simulink model "old_SMC"  (R2023a)
settings: Solver=FixedStepAuto  StartTime=0.0  StopTime=inf  RelTol=1e-3
undefined symbols (not defined in the file or in its folder): angular, linear
libraries: ros2lib x24
(part 1 of 2)

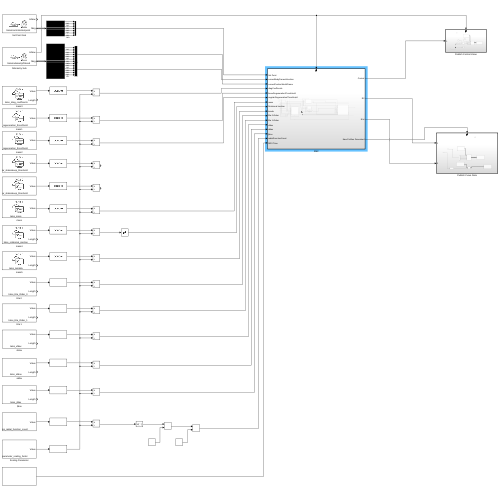
[thumbnail: Simulink's stored preview of the top-level diagram]
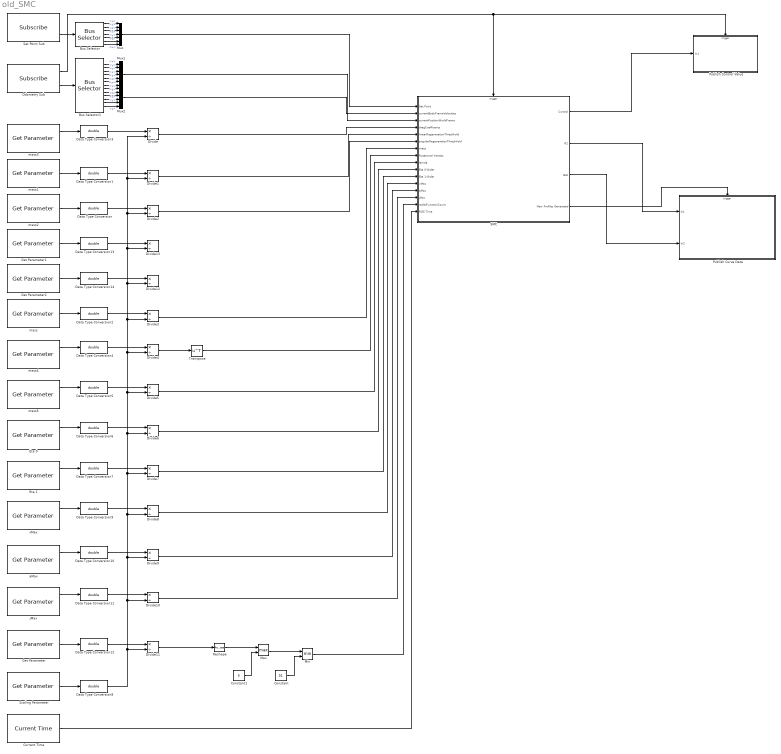
== system old_SMC ==
  Bus Selector : BusSelector  OutputSignals=position.x,position.y,position.z,orientation.x,orientation.y,orientation.z,orientation.w
  Bus Selector1 : BusSelector  OutputSignals=pose.pose.position.x,pose.pose.position.y,pose.pose.position.z,pose.pose.orientation.x,pose.pose.orientation.y,pose.pose.orientation.z,pose.pose.orientation.w,twist.twist.linear.x,twist.twist.linear.y,twist.twist.linear.z,twist.twist.angular.x,twist.twist.angular.y,twist.twist.angular.z
  Constant : Constant  Value=51
  Constant1 : Constant  Value=5
  Current Time : ros2lib/Current Time  OutputFormat=double  SampleTime=-1  ModelName=SMC
  Data Type Conversion{,1..14} (15 alike) : DataTypeConversion  OutDataTypeStr=double  SaturateOnIntegerOverflow=off  RndMeth=Floor
  Divide{,1..13} (14 alike) : Product  Inputs=*/
  Eta 0 : ros2lib/Get Parameter  ParameterName=talos_Eta_Order_0  ParameterType=int64[]  ParameterMaxArrayLength=6  ParameterInitialValue=0.0  SampleTime=-1  ModelName=SMC  BlockId=ParamGet_SMC_204
  Eta 1 : ros2lib/Get Parameter  ParameterName=talos_Eta_Order_1  ParameterType=int64[]  ParameterMaxArrayLength=6  ParameterInitialValue=0.0  SampleTime=-1  ModelName=SMC  BlockId=ParamGet_SMC_206
  Get Parameter : ros2lib/Get Parameter  ParameterName=talos_radial_function_count  ParameterType=int64  ParameterMaxArrayLength=16  ParameterInitialValue=0.0  SampleTime=-1  ModelName=SMC  BlockId=ParamGet_SMC_267
  Get Parameter1 : ros2lib/Get Parameter  ParameterName=talos_angular_stationkeep_threshold  ParameterType=int64  ParameterMaxArrayLength=16  ParameterInitialValue=0.0  SampleTime=-1  ModelName=SMC  BlockId=ParamGet_SMC_367
  Get Parameter2 : ros2lib/Get Parameter  ParameterName=talos_linear_stationkeep_threshold  ParameterType=int64  ParameterMaxArrayLength=16  ParameterInitialValue=0.0  SampleTime=-1  ModelName=SMC  BlockId=ParamGet_SMC_368
  Max : MinMax  Function=max  Inputs=2
  Min : MinMax  Inputs=2
  Mux : Mux  Inputs=7
  Mux1 : Mux  Inputs=7
  Mux2 : Mux  Inputs=6
  Odometry Sub : ros2lib/Subscribe  topicSource=Specify your own  topic=/talos/odometry/filtered  messageType=nav_msgs/Odometry  sampleTime=-1  QOSHistory=Keep last  QOSDepth=1  QOSReliability=Reliable  QOSDurability=Volatile
  Publish Control Value : Subsystem
  Publish Curve Data : Subsystem
  Reshape : Reshape  OutputDimensions=1
  SMC : Subsystem
  Scaling Parameter : ros2lib/Get Parameter  ParameterName=parameter_scaling_factor  ParameterType=int64  ParameterMaxArrayLength=16  ParameterInitialValue=1000000  SampleTime=-1  ModelName=SMC  BlockId=ParamGet_SMC_208
  Set Point Sub : ros2lib/Subscribe  topicSource=Specify your own  topic=/talos/controller/setpoint  messageType=geometry_msgs/Pose  sampleTime=-1  QOSHistory=Keep last  QOSDepth=1  QOSReliability=Reliable  QOSDurability=Volatile
  Transpose : Math  Operator=transpose
  aMax : ros2lib/Get Parameter  ParameterName=talos_aMax  ParameterType=int64[]  ParameterMaxArrayLength=6  ParameterInitialValue=0.0  SampleTime=-1  ModelName=SMC  BlockId=ParamGet_SMC_242
  jMax : ros2lib/Get Parameter  ParameterName=talos_jMax  ParameterType=int64[]  ParameterMaxArrayLength=6  ParameterInitialValue=0.0  SampleTime=-1  ModelName=SMC  BlockId=ParamGet_SMC_244
  mass : ros2lib/Get Parameter  ParameterName=talos_mass  ParameterType=int64  ParameterMaxArrayLength=16  ParameterInitialValue=0.0  SampleTime=-1  ModelName=SMC  BlockId=ParamGet_SMC_190
  mass1 : ros2lib/Get Parameter  ParameterName=talos_angular_regeneration_threshhold  ParameterType=int64  ParameterMaxArrayLength=16  ParameterInitialValue=0.0  SampleTime=-1  ModelName=SMC  BlockId=ParamGet_SMC_192
  mass2 : ros2lib/Get Parameter  ParameterName=talos_linear_regeneration_threshhold  ParameterType=int64  ParameterMaxArrayLength=16  ParameterInitialValue=0.0  SampleTime=-1  ModelName=SMC  BlockId=ParamGet_SMC_193
  mass3 : ros2lib/Get Parameter  ParameterName=talos_drag_coefficents  ParameterType=int64[]  ParameterMaxArrayLength=24  ParameterInitialValue=0.0  SampleTime=-1  ModelName=SMC  BlockId=ParamGet_SMC_197
  mass4 : ros2lib/Get Parameter  ParameterName=talos_rotational_inertias  ParameterType=int64[]  ParameterMaxArrayLength=3  ParameterInitialValue=0.0  SampleTime=-1  ModelName=SMC  BlockId=ParamGet_SMC_199
  mass5 : ros2lib/Get Parameter  ParameterName=talos_lambda  ParameterType=int64[]  ParameterMaxArrayLength=6  ParameterInitialValue=0.0  SampleTime=-1  ModelName=SMC  BlockId=ParamGet_SMC_202
  vMax : ros2lib/Get Parameter  ParameterName=talos_vMax  ParameterType=int64[]  ParameterMaxArrayLength=6  ParameterInitialValue=0.0  SampleTime=-1  ModelName=SMC  BlockId=ParamGet_SMC_240
  wires:
  Set Point Sub/2 -> Bus Selector/1
  Bus Selector/1 -> Mux/1  "<x>"
  Bus Selector/2 -> Mux/2  "<y>"
  Bus Selector/3 -> Mux/3  "<z>"
  Bus Selector/4 -> Mux/4  "<x>"
  Bus Selector/5 -> Mux/5  "<y>"
  Bus Selector/7 -> Mux/7  "<w>"
  Bus Selector/6 -> Mux/6  "<z>"
  Mux/1 -> SMC/1(Set Point)
  Odometry Sub/2 -> Bus Selector1/1
  Bus Selector1/1 -> Mux1/1  "<x>"
  Bus Selector1/2 -> Mux1/2  "<y>"
  Bus Selector1/3 -> Mux1/3  "<z>"
  Bus Selector1/4 -> Mux1/4  "<x>"
  Bus Selector1/5 -> Mux1/5  "<y>"
  Bus Selector1/6 -> Mux1/6  "<z>"
  Bus Selector1/7 -> Mux1/7  "<w>"
  Bus Selector1/8 -> Mux2/1  "<x>"
  Bus Selector1/9 -> Mux2/2  "<y>"
  Bus Selector1/10 -> Mux2/3  "<z>"
  Bus Selector1/11 -> Mux2/4  "<x>"
  Bus Selector1/12 -> Mux2/5  "<y>"
  Bus Selector1/13 -> Mux2/6  "<z>"
  Mux1/1 -> SMC/3(currentPositionWorldFrame)
  Mux2/1 -> SMC/2(currentBodyFrameVelocities)
  mass2/1 -> Data Type Conversion/1
  mass/1 -> Data Type Conversion2/1
  mass1/1 -> Data Type Conversion1/1
  mass3/1 -> Data Type Conversion3/1
  mass4/1 -> Data Type Conversion4/1
  mass5/1 -> Data Type Conversion5/1
  Eta 0/1 -> Data Type Conversion6/1
  Eta 1/1 -> Data Type Conversion7/1
  Scaling Parameter/1 -> Data Type Conversion8/1
  Data Type Conversion3/1 -> Divide/1
  Data Type Conversion1/1 -> Divide1/1
  Data Type Conversion/1 -> Divide2/1
  Data Type Conversion2/1 -> Divide3/1
  Data Type Conversion4/1 -> Divide4/1
  Data Type Conversion5/1 -> Divide5/1
  Data Type Conversion6/1 -> Divide6/1
  Data Type Conversion7/1 -> Divide7/1
  Data Type Conversion8/1 -> Divide11/2, Divide10/2, Divide9/2, Divide8/2, Divide7/2, Divide6/2, Divide5/2, Divide4/2, Divide3/2, Divide12/2, Divide13/2, Divide2/2, Divide1/2, Divide/2
  Divide/1 -> SMC/4(dragCoefficents)
  Divide1/1 -> SMC/5(linearRegenerationThreshhold)
  Divide2/1 -> SMC/6(angularRegenerationThreshhold)
  Divide3/1 -> SMC/7(mass)
  Divide4/1 -> Transpose/1
  Divide5/1 -> SMC/9(lamda)
  Divide6/1 -> SMC/10(Eta 0-Order)
  Divide7/1 -> SMC/11(Eta 1-Order)
  vMax/1 -> Data Type Conversion9/1
  aMax/1 -> Data Type Conversion10/1
  jMax/1 -> Data Type Conversion11/1
  Data Type Conversion9/1 -> Divide8/1
  Data Type Conversion10/1 -> Divide9/1
  Data Type Conversion11/1 -> Divide10/1
  Divide8/1 -> SMC/12(vMax)
  Divide9/1 -> SMC/13(aMax)
  Divide10/1 -> SMC/14(jMax)
  SMC/2(R2) -> Publish Curve Data/1(In1)
  SMC/3(tEst) -> Publish Curve Data/2(In2)
  SMC/4(New Profiles Generated) -> Publish Curve Data/Trigger
  Transpose/1 -> SMC/8(Rotational Inertias)
  Get Parameter/1 -> Data Type Conversion12/1
  Data Type Conversion12/1 -> Divide11/1
  Divide11/1 -> Reshape/1
  Constant/1 -> Min/2
  Min/1 -> SMC/15(radialFunctionCount)
  Current Time/1 -> SMC/16(ROS Time)
  Reshape/1 -> Max/1
  Max/1 -> Min/1
  Constant1/1 -> Max/2
  Get Parameter1/1 -> Data Type Conversion13/1
  Get Parameter2/1 -> Data Type Conversion14/1
  Data Type Conversion14/1 -> Divide12/1
  Data Type Conversion13/1 -> Divide13/1
  SMC/1(Control) -> Publish Control Value/1(In1)
  Odometry Sub/1 -> SMC/Trigger, Publish Control Value/Trigger

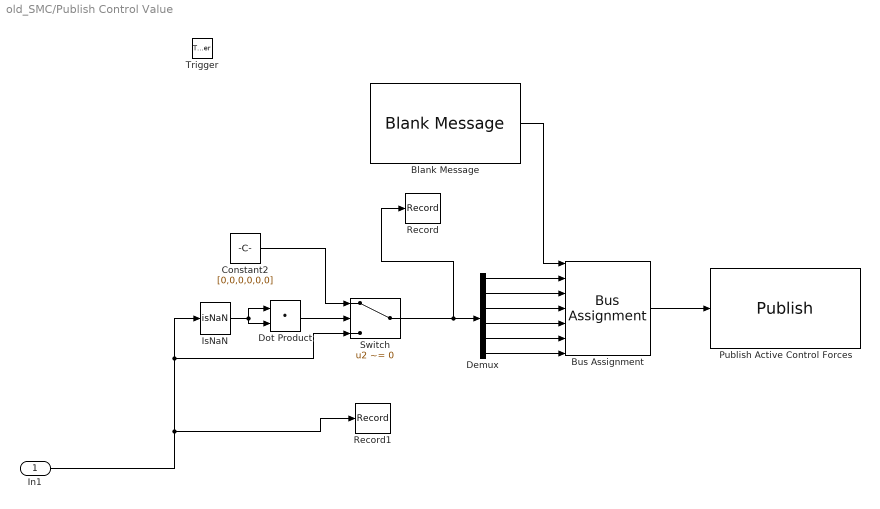
== system old_SMC/Publish Control Value ==
  In1 : Inport
  Trigger : TriggerPort  VariantControl=(inherit)  PortDimensions=1
  Blank Message : ros2lib/Blank Message  messageClass=Message  entityType=geometry_msgs/Twist  messageType=geometry_msgs/Twist  SampleTime=inf
  Bus Assignment : BusAssignment  AssignedSignals=linear.x,linear.y,linear.z,angular.x,angular.y,angular.z
  Constant2 : Constant  Value=[0,0,0,0,0,0]
  Demux : Demux  Outputs=6
  Dot Product : DotProduct  OutDataTypeStr=Inherit: Inherit via internal rule
  IsNaN : RelationalOperator  Operator=isNaN  OutDataTypeStr=boolean  RndMeth=Simplest  InputSameDT=off
  Publish Active Control Forces : ros2lib/Publish  topicSource=Specify your own  topic=/talos/controller/active_body_force  messageType=geometry_msgs/Twist  QOSHistory=Keep last  QOSDepth=1  QOSReliability=Reliable  QOSDurability=Volatile
  Record : Record  FileSettingsInternal="{\"entries\":[{\"content\":{\"excelSettings\":{\"content\":{},\"type\":\"Streamout.ExcelSettings\"}},\"type\":\"Streamout.FileSettingStorage\",\"uuid\":\"\"}],\"packageUris\":[\"http:\\/\\/schema.mathworks.com\\/mf0\\/streamout_blocks\\/R2020a\"],\"version\":\"1.0\"}"  Layout=[1 1]  SignalsInternal="{\"entries\":[{\"content\":{\"signals\":[{\"content\":{\"blockPath\":[],\"dimensions\":[6],\"domain\":\"\",\"hasChildren\":true,\"lineColor\":\"#d95319\",\"port\":1,\"sid\":[\"\"],\"signalID\":32364,\"signalName\":\"Switch\"},\"type\":\"RecordBlkView.Signal\",\"uuid\":\"\"},{\"content\":{\"blockPath\":[],\"channel\":[1],\"dimensions\":[6],\"domain\":\"\",\"lineColor\":\"#77ac30\",\"parentID\":32364,\"port\":1,\"sid\":[\"\"],\"signalID\":32365,\"signalName\":\"Switch\" ...(+1250 chars)"  VisualizationBindings="{\"sparklinesplugin\":{\"info\":[{\"bindingParametersList\":[],\"subplotID\":1}]}}"
  Record1 : Record  FileSettingsInternal="{\"entries\":[{\"content\":{\"excelSettings\":{\"content\":{},\"type\":\"Streamout.ExcelSettings\"}},\"type\":\"Streamout.FileSettingStorage\",\"uuid\":\"\"}],\"packageUris\":[\"http:\\/\\/schema.mathworks.com\\/mf0\\/streamout_blocks\\/R2020a\"],\"version\":\"1.0\"}"  Layout=[1 1]  SignalsInternal="{\"entries\":[{\"content\":{\"signals\":[{\"content\":{\"blockPath\":[],\"dimensions\":[6],\"domain\":\"\",\"hasChildren\":true,\"lineColor\":\"#7e2f8e\",\"port\":1,\"sid\":[\"\"],\"signalID\":32369,\"signalName\":\"In1\"},\"type\":\"RecordBlkView.Signal\",\"uuid\":\"\"},{\"content\":{\"blockPath\":[],\"channel\":[1],\"dimensions\":[6],\"domain\":\"\",\"lineColor\":\"#22b573\",\"parentID\":32369,\"plots\":[1],\"port\":1,\"sid\":[\"\"],\"signalID\":32370,\"signalName\" ...(+1289 chars)"  VisualizationBindings="{\"sparklinesplugin\":{\"info\":[{\"bindingParametersList\":[],\"subplotID\":1}]}}"
  Switch : Switch  Criteria=u2 ~= 0  SaturateOnIntegerOverflow=off  InputSameDT=off
  wires:
  Blank Message/1 -> Bus Assignment/1
  Switch/1 -> Record/1, Demux/1
  IsNaN/1 -> Dot Product/1, Dot Product/2
  Constant2/1 -> Switch/1
  Dot Product/1 -> Switch/2
  Demux/1 -> Bus Assignment/2
  Demux/2 -> Bus Assignment/3
  Demux/6 -> Bus Assignment/7
  Demux/3 -> Bus Assignment/4
  Demux/5 -> Bus Assignment/6
  In1/1 -> Record1/1, IsNaN/1, Switch/3
  Demux/4 -> Bus Assignment/5
  Bus Assignment/1 -> Publish Active Control Forces/1

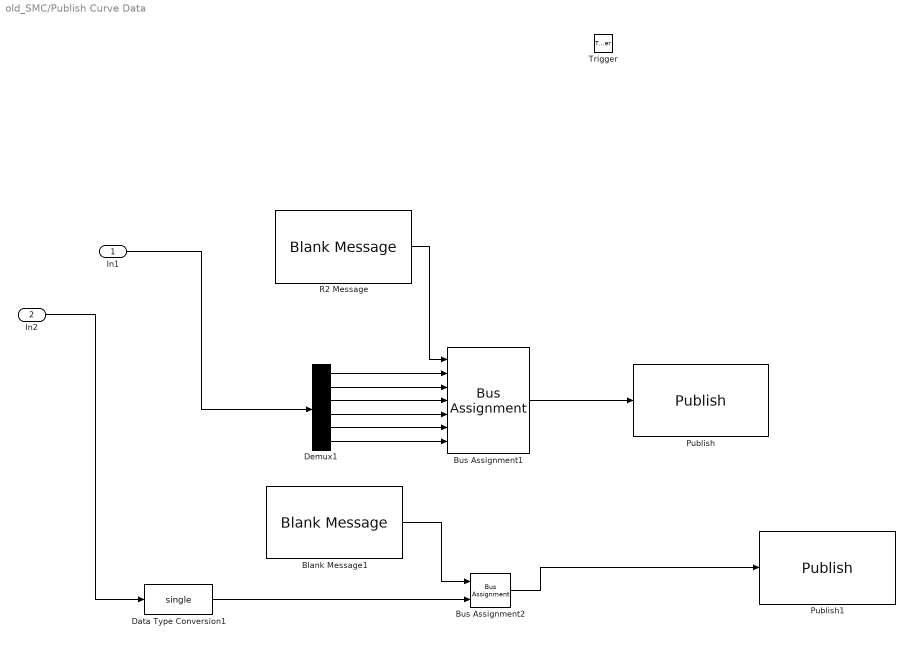
== system old_SMC/Publish Curve Data ==
  In1 : Inport
  In2 : Inport  Port=2
  Trigger : TriggerPort  VariantControl=(inherit)  PortDimensions=1
  Blank Message1 : ros2lib/Blank Message  messageClass=Message  entityType=std_msgs/Float32  messageType=std_msgs/Float32  SampleTime=inf
  Bus Assignment1 : BusAssignment  AssignedSignals=linear.x,angular.x,angular.y,angular.z,linear.y,linear.z
  Bus Assignment2 : BusAssignment  AssignedSignals=data
  Data Type Conversion1 : DataTypeConversion  OutDataTypeStr=single  SaturateOnIntegerOverflow=off  RndMeth=Floor
  Demux1 : Demux  Outputs=6
  Publish : ros2lib/Publish  topicSource=Specify your own  topic=/talos/controller/generatedR2  messageType=geometry_msgs/Twist  QOSHistory=Keep last  QOSDepth=1  QOSReliability=Reliable  QOSDurability=Volatile
  Publish1 : ros2lib/Publish  topicSource=Specify your own  topic=/talos/controller/curveTime  messageType=std_msgs/Float32  QOSHistory=Keep last  QOSDepth=1  QOSReliability=Reliable  QOSDurability=Volatile
  R2 Message : ros2lib/Blank Message  messageClass=Message  entityType=geometry_msgs/Twist  messageType=geometry_msgs/Twist  SampleTime=inf
  wires:
  Demux1/1 -> Bus Assignment1/2
  Demux1/6 -> Bus Assignment1/7
  Blank Message1/1 -> Bus Assignment2/1
  R2 Message/1 -> Bus Assignment1/1
  Demux1/5 -> Bus Assignment1/6
  Demux1/3 -> Bus Assignment1/4
  Demux1/4 -> Bus Assignment1/5
  Bus Assignment1/1 -> Publish/1
  In2/1 -> Data Type Conversion1/1
  Demux1/2 -> Bus Assignment1/3
  Bus Assignment2/1 -> Publish1/1
  In1/1 -> Demux1/1
  Data Type Conversion1/1 -> Bus Assignment2/2

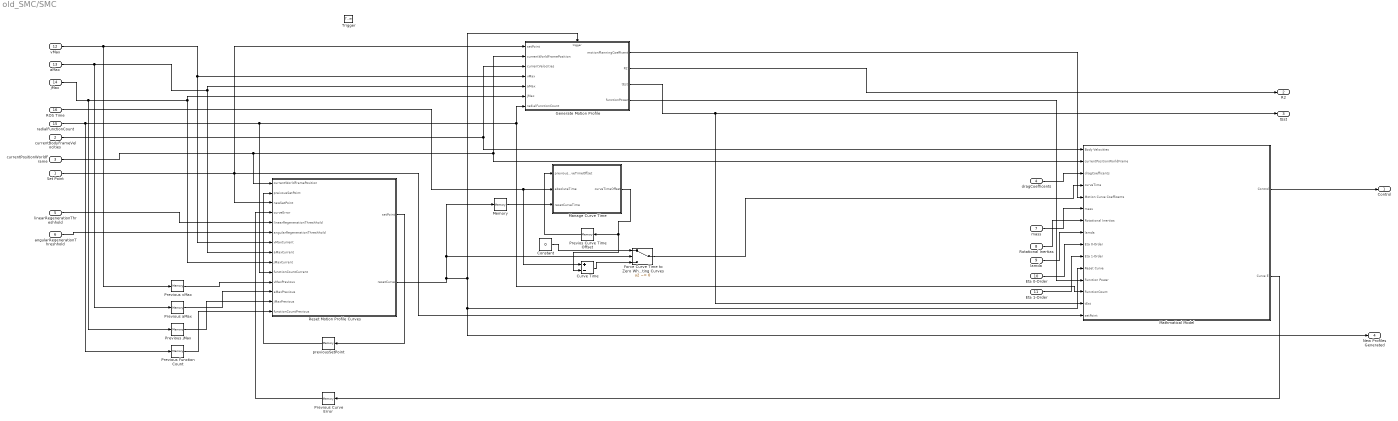
== system old_SMC/SMC ==
  Set Point : Inport
  currentBodyFrameVelocities : Inport  Port=2
  currentPositionWorldFrame : Inport  Port=3
  dragCoefficents : Inport  Port=4
  linearRegenerationThreshhold : Inport  Port=5
  angularRegenerationThreshhold : Inport  Port=6
  mass : Inport  Port=7
  Rotational Inertias : Inport  Port=8
  lamda : Inport  Port=9
  Eta 0-Order : Inport  Port=10
  Eta 1-Order : Inport  Port=11
  vMax : Inport  Port=12
  aMax : Inport  Port=13
  jMax : Inport  Port=14
  radialFunctionCount : Inport  Port=15
  ROS Time : Inport  Port=16
  Trigger : TriggerPort  VariantControl=(inherit)  PortDimensions=1
  Constant : Constant  Value=0
  Curve Time : Sum  Inputs=+-
  Force Curve Time to Zero When Reseting Curves : Switch  Criteria=u2 ~= 0  SaturateOnIntegerOverflow=off  InputSameDT=off
  Generate Motion Profile : Subsystem
  Manage Curve Time : MATLAB Function  TreatAsAtomicUnit=on
  Mathmatical Model : Subsystem
  Memory : Memory  InheritSampleTime=on
  Previos Curve Time Offset : Memory  InitialCondition=1700540270  InheritSampleTime=on
  Previous Curve Error : Memory  InheritSampleTime=on
  Previous Function Count : Memory  InheritSampleTime=on
  Previous aMax : Memory  InheritSampleTime=on
  Previous jMax : Memory  InheritSampleTime=on
  Previous vMax : Memory  InheritSampleTime=on
  Reset Motion Profile Curves : MATLAB Function  TreatAsAtomicUnit=on
  previousSetPoint : Memory  InheritSampleTime=on
  Control : Outport
  R2 : Outport  Port=2
  tEst : Outport  Port=3
  New Profiles Generated : Outport  Port=4
  wires:
  lamda/1 -> Mathmatical Model/8(lamda)
  currentPositionWorldFrame/1 -> Reset Motion Profile Curves/1(currentWorldFramePosition), Generate Motion Profile/2(currentWorldFramePosition), Mathmatical Model/2(currentPositionWorldFrame)
  mass/1 -> Mathmatical Model/6(mass)
  previousSetPoint/1 -> Reset Motion Profile Curves/2(preivousSetPoint)
  Mathmatical Model/2(Curve E) -> Previous Curve Error/1
  Rotational Inertias/1 -> Mathmatical Model/7(Rotational Inertias)
  currentBodyFrameVelocities/1 -> Generate Motion Profile/3(currentVelocities), Mathmatical Model/1(Body Velocities)
  Eta 0-Order/1 -> Mathmatical Model/9(Eta 0-Order)
  Eta 1-Order/1 -> Mathmatical Model/10(Eta 1-Order)
  dragCoefficents/1 -> Mathmatical Model/3(dragCoefficents)
  angularRegenerationThreshhold/1 -> Reset Motion Profile Curves/6(angularRegenerationThreshhold)
  linearRegenerationThreshhold/1 -> Reset Motion Profile Curves/5(linearRegenerationThreshhold)
  Previous Curve Error/1 -> Reset Motion Profile Curves/4(curveError)
  Reset Motion Profile Curves/1(setPoint) -> previousSetPoint/1
  Generate Motion Profile/1(motionPlanningCoefficents) -> Mathmatical Model/5(Motion Curve Coefficents)
  Generate Motion Profile/2(R2) -> R2/1
  Generate Motion Profile/3(tEst) -> Mathmatical Model/14(tEst), tEst/1
  vMax/1 -> Previous vMax/1, Reset Motion Profile Curves/7(vMaxCurrent), Generate Motion Profile/4(vMax)
  aMax/1 -> Previous aMax/1, Reset Motion Profile Curves/8(aMaxCurrent), Generate Motion Profile/5(aMax)
  jMax/1 -> Previous jMax/1, Reset Motion Profile Curves/9(jMaxCurrent), Generate Motion Profile/6(jMax)
  radialFunctionCount/1 -> Previous Function Count/1, Reset Motion Profile Curves/10(functionCountCurrent), Mathmatical Model/13(FunctionCount), Generate Motion Profile/7(radialFunctionCount)
  Generate Motion Profile/4(functionPower) -> Mathmatical Model/12(Function Power)
  Previous Function Count/1 -> Reset Motion Profile Curves/14(functionCountPrevious)
  Previous jMax/1 -> Reset Motion Profile Curves/13(jMaxPrevious)
  Previous aMax/1 -> Reset Motion Profile Curves/12(aMaxPrevious)
  Previous vMax/1 -> Reset Motion Profile Curves/11(vMaxPrevious)
  Reset Motion Profile Curves/2(resetCurve) -> Memory/1, Force Curve Time to Zero When Reseting Curves/2, New Profiles Generated/1, Mathmatical Model/11(Reset Curve), Generate Motion Profile/Trigger
  ROS Time/1 -> Curve Time/1, Manage Curve Time/2(absoluteTime)
  Manage Curve Time/1(curveTimeOffset) -> Curve Time/2, Previos Curve Time Offset/1
  Previos Curve Time Offset/1 -> Manage Curve Time/1(previousCurveTimeOffset)
  Memory/1 -> Manage Curve Time/3(resetCurveTime)
  Curve Time/1 -> Force Curve Time to Zero When Reseting Curves/3
  Force Curve Time to Zero When Reseting Curves/1 -> Mathmatical Model/4(curveTime)
  Constant/1 -> Force Curve Time to Zero When Reseting Curves/1
  Set Point/1 -> Mathmatical Model/15(setPoint), Reset Motion Profile Curves/3(newSetPoint), Generate Motion Profile/1(setPoint)
  Mathmatical Model/1(Control) -> Control/1

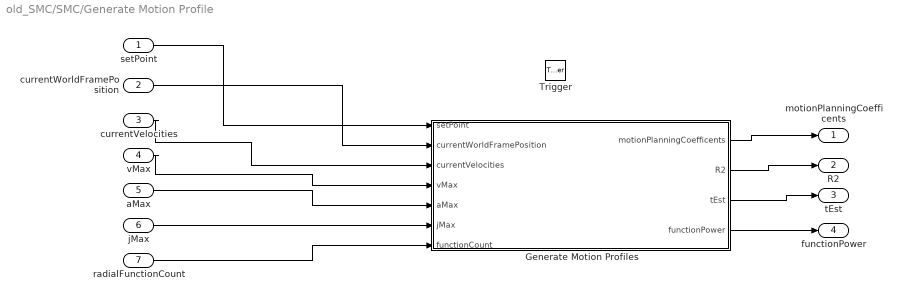
== system old_SMC/SMC/Generate Motion Profile ==
  setPoint : Inport
  currentWorldFramePosition : Inport  Port=2
  currentVelocities : Inport  Port=3
  vMax : Inport  Port=4
  aMax : Inport  Port=5
  jMax : Inport  Port=6
  radialFunctionCount : Inport  Port=7
  Trigger : TriggerPort  VariantControl=(inherit)  InitialTriggerSignalState=zero  PortDimensions=1
  Generate Motion Profiles : MATLAB Function  TreatAsAtomicUnit=on
  motionPlanningCoefficents : Outport
  R2 : Outport  Port=2
  tEst : Outport  Port=3
  functionPower : Outport  Port=4
  wires:
  Generate Motion Profiles/2(R2) -> R2/1
  currentVelocities/1 -> Generate Motion Profiles/3(currentVelocities)
  Generate Motion Profiles/1(motionPlanningCoefficents) -> motionPlanningCoefficents/1
  Generate Motion Profiles/3(tEst) -> tEst/1
  setPoint/1 -> Generate Motion Profiles/1(setPoint)
  aMax/1 -> Generate Motion Profiles/5(aMax)
  vMax/1 -> Generate Motion Profiles/4(vMax)
  currentWorldFramePosition/1 -> Generate Motion Profiles/2(currentWorldFramePosition)
  jMax/1 -> Generate Motion Profiles/6(jMax)
  radialFunctionCount/1 -> Generate Motion Profiles/7(functionCount)
  Generate Motion Profiles/4(functionPower) -> functionPower/1

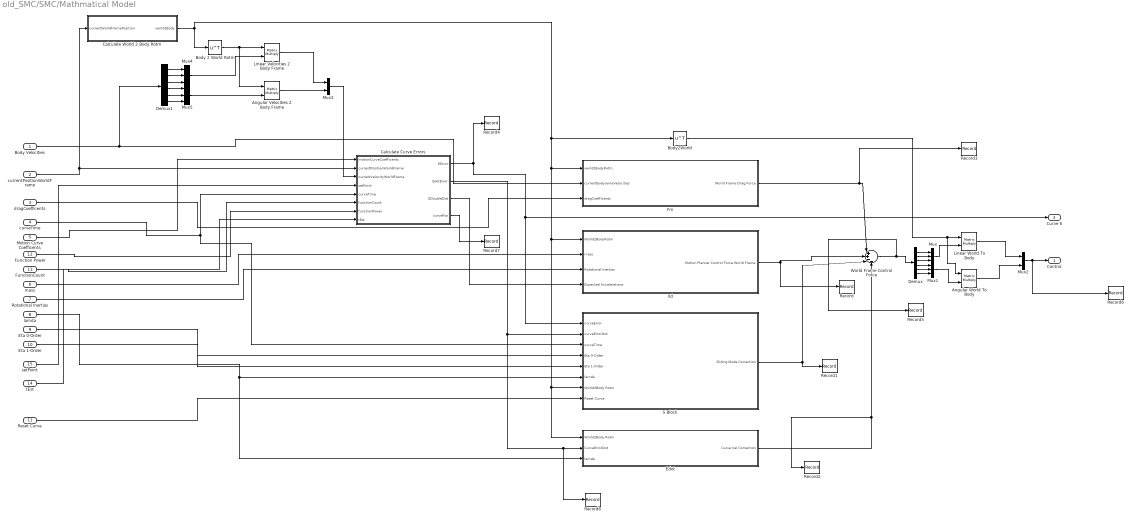
== system old_SMC/SMC/Mathmatical Model ==
  Body Velocities : Inport
  currentPositionWorldFrame : Inport  Port=2
  dragCoefficents : Inport  Port=3
  curveTime : Inport  Port=4
  Motion Curve Coefficents : Inport  Port=5
  mass : Inport  Port=6
  Rotational Inertias : Inport  Port=7
  lamda : Inport  Port=8
  Eta 0-Order : Inport  Port=9
  Eta 1-Order : Inport  Port=10
  Reset Curve : Inport  Port=11
  Function Power : Inport  Port=12
  FunctionCount : Inport  Port=13
  tEst : Inport  Port=14
  setPoint : Inport  Port=15
  Angular Velocities 2 Body Frame : Product  Multiplication=Matrix(*)
  Angular World To Body : Product  Multiplication=Matrix(*)
  Body 2 World Rotm : Math  Operator=transpose
  Body2World : Math  Operator=transpose
  Calculate Curve Errors : MATLAB Function  TreatAsAtomicUnit=on
  Calculate World 2 Body Rotm : MATLAB Function  TreatAsAtomicUnit=on
  Demux : Demux  Outputs=6
  Demux1 : Demux  Outputs=6
  Edot : Subsystem
  Fm : Subsystem
  Linear Velocities 2 Body Frame : Product  Multiplication=Matrix(*)
  Linear World To Body : Product  Multiplication=Matrix(*)
  Mux{,1,4..5} (4 alike) : Mux  Inputs=3
  Mux2 : Mux  Inputs=2
  Mux3 : Mux  Inputs=2
  Record : Record  FileSettingsInternal="{\"entries\":[{\"content\":{\"excelSettings\":{\"content\":{},\"type\":\"Streamout.ExcelSettings\"}},\"type\":\"Streamout.FileSettingStorage\",\"uuid\":\"\"}],\"packageUris\":[\"http:\\/\\/schema.mathworks.com\\/mf0\\/streamout_blocks\\/R2020a\"],\"version\":\"1.0\"}"  Layout=[1 1]  SignalsInternal="{\"entries\":[{\"content\":{\"signals\":[{\"content\":{\"blockPath\":[],\"dimensions\":[6,1],\"domain\":\"\",\"hasChildren\":true,\"lineColor\":\"#139fff\",\"port\":1,\"sid\":[\"\"],\"signalID\":32309,\"signalName\":\"Xd\"},\"type\":\"RecordBlkView.Signal\",\"uuid\":\"\"},{\"content\":{\"blockPath\":[],\"channel\":[1,1],\"dimensions\":[6,1],\"domain\":\"\",\"lineColor\":\"#fe330a\",\"parentID\":32309,\"plots\":[1],\"port\":1,\"sid\":[\"\"],\"signalID\":32310,\"signal ...(+1308 chars)"  VisualizationBindings="{\"sparklinesplugin\":{\"info\":[{\"bindingParametersList\":[],\"subplotID\":1}]}}"
  Record1 : Record  FileSettingsInternal="{\"entries\":[{\"content\":{\"excelSettings\":{\"content\":{},\"type\":\"Streamout.ExcelSettings\"}},\"type\":\"Streamout.FileSettingStorage\",\"uuid\":\"\"}],\"packageUris\":[\"http:\\/\\/schema.mathworks.com\\/mf0\\/streamout_blocks\\/R2020a\"],\"version\":\"1.0\"}"  Layout=[1 1]  SignalsInternal="{\"entries\":[{\"content\":{\"signals\":[{\"content\":{\"blockPath\":[],\"dimensions\":[6,1],\"domain\":\"\",\"hasChildren\":true,\"lineColor\":\"#b746ff\",\"port\":1,\"sid\":[\"\"],\"signalID\":32314,\"signalName\":\"S Block\"},\"type\":\"RecordBlkView.Signal\",\"uuid\":\"\"},{\"content\":{\"blockPath\":[],\"channel\":[1,1],\"dimensions\":[6,1],\"domain\":\"\",\"lineColor\":\"#0072bd\",\"parentID\":32314,\"plots\":[1],\"port\":1,\"sid\":[\"\"],\"signalID\":32315,\"s ...(+1343 chars)"  VisualizationBindings="{\"sparklinesplugin\":{\"info\":[{\"bindingParametersList\":[],\"subplotID\":1}]}}"
  Record2 : Record  FileSettingsInternal="{\"entries\":[{\"content\":{\"excelSettings\":{\"content\":{},\"type\":\"Streamout.ExcelSettings\"}},\"type\":\"Streamout.FileSettingStorage\",\"uuid\":\"\"}],\"packageUris\":[\"http:\\/\\/schema.mathworks.com\\/mf0\\/streamout_blocks\\/R2020a\"],\"version\":\"1.0\"}"  Layout=[1 1]  SignalsInternal="{\"entries\":[{\"content\":{\"signals\":[{\"content\":{\"blockPath\":[],\"dimensions\":[6,1],\"domain\":\"\",\"hasChildren\":true,\"lineColor\":\"#ff13a6\",\"port\":1,\"sid\":[\"\"],\"signalID\":32319,\"signalName\":\"Edot\"},\"type\":\"RecordBlkView.Signal\",\"uuid\":\"\"},{\"content\":{\"blockPath\":[],\"channel\":[1,1],\"dimensions\":[6,1],\"domain\":\"\",\"lineColor\":\"#edb120\",\"parentID\":32319,\"port\":1,\"sid\":[\"\"],\"signalID\":32320,\"signalName\":\"Edo ...(+1298 chars)"  VisualizationBindings="{\"sparklinesplugin\":{\"info\":[{\"bindingParametersList\":[],\"subplotID\":1}]}}"
  Record3 : Record  FileSettingsInternal="{\"entries\":[{\"content\":{\"excelSettings\":{\"content\":{},\"type\":\"Streamout.ExcelSettings\"}},\"type\":\"Streamout.FileSettingStorage\",\"uuid\":\"\"}],\"packageUris\":[\"http:\\/\\/schema.mathworks.com\\/mf0\\/streamout_blocks\\/R2020a\"],\"version\":\"1.0\"}"  Layout=[1 1]  SignalsInternal="{\"entries\":[{\"content\":{\"signals\":[{\"content\":{\"blockPath\":[],\"dimensions\":[6],\"domain\":\"\",\"hasChildren\":true,\"lineColor\":\"#22b573\",\"port\":1,\"sid\":[\"\"],\"signalID\":32324,\"signalName\":\"Fm\"},\"type\":\"RecordBlkView.Signal\",\"uuid\":\"\"},{\"content\":{\"blockPath\":[],\"channel\":[1],\"dimensions\":[6],\"domain\":\"\",\"lineColor\":\"#77ac30\",\"parentID\":32324,\"plots\":[1],\"port\":1,\"sid\":[\"\"],\"signalID\":32325,\"signalName\": ...(+1246 chars)"  VisualizationBindings="{\"sparklinesplugin\":{\"info\":[{\"bindingParametersList\":[],\"subplotID\":1}]}}"
  Record4 : Record  FileSettingsInternal="{\"entries\":[{\"content\":{\"excelSettings\":{\"content\":{},\"type\":\"Streamout.ExcelSettings\"}},\"type\":\"Streamout.FileSettingStorage\",\"uuid\":\"\"}],\"packageUris\":[\"http:\\/\\/schema.mathworks.com\\/mf0\\/streamout_blocks\\/R2020a\"],\"version\":\"1.0\"}"  Layout=[1 1]  SignalsInternal="{\"entries\":[{\"content\":{\"signals\":[{\"content\":{\"blockPath\":[],\"dimensions\":[6,1],\"domain\":\"\",\"hasChildren\":true,\"lineColor\":\"#d95319\",\"port\":1,\"sid\":[\"\"],\"signalID\":32329,\"signalName\":\"Calculate Curve Errors:1\"},\"type\":\"RecordBlkView.Signal\",\"uuid\":\"\"},{\"content\":{\"blockPath\":[],\"channel\":[1,1],\"dimensions\":[6,1],\"domain\":\"\",\"lineColor\":\"#a2142f\",\"parentID\":32329,\"plots\":[1],\"port\":1,\"sid\":[\"\"],\"s ...(+1462 chars)"  VisualizationBindings="{\"sparklinesplugin\":{\"info\":[{\"bindingParametersList\":[],\"subplotID\":1}]}}"
  Record5 : Record  FileSettingsInternal="{\"entries\":[{\"content\":{\"excelSettings\":{\"content\":{},\"type\":\"Streamout.ExcelSettings\"}},\"type\":\"Streamout.FileSettingStorage\",\"uuid\":\"\"}],\"packageUris\":[\"http:\\/\\/schema.mathworks.com\\/mf0\\/streamout_blocks\\/R2020a\"],\"version\":\"1.0\"}"  Layout=[1 1]  SignalsInternal="{\"entries\":[{\"content\":{\"signals\":[{\"content\":{\"blockPath\":[],\"dimensions\":[6,1],\"domain\":\"\",\"hasChildren\":true,\"lineColor\":\"#7e2f8e\",\"port\":1,\"sid\":[\"\"],\"signalID\":32334,\"signalName\":\"World Frame Control Force\"},\"type\":\"RecordBlkView.Signal\",\"uuid\":\"\"},{\"content\":{\"blockPath\":[],\"channel\":[1,1],\"dimensions\":[6,1],\"domain\":\"\",\"lineColor\":\"#4dbeee\",\"parentID\":32334,\"port\":1,\"sid\":[\"\"],\"signalID\":32 ...(+1409 chars)"  VisualizationBindings="{\"sparklinesplugin\":{\"info\":[{\"bindingParametersList\":[],\"subplotID\":1}]}}"
  Record6 : Record  FileSettingsInternal="{\"entries\":[{\"content\":{\"excelSettings\":{\"content\":{},\"type\":\"Streamout.ExcelSettings\"}},\"type\":\"Streamout.FileSettingStorage\",\"uuid\":\"\"}],\"packageUris\":[\"http:\\/\\/schema.mathworks.com\\/mf0\\/streamout_blocks\\/R2020a\"],\"version\":\"1.0\"}"  Layout=[1 1]  SignalsInternal="{\"entries\":[{\"content\":{\"signals\":[{\"content\":{\"blockPath\":[],\"dimensions\":[6],\"domain\":\"\",\"hasChildren\":true,\"lineColor\":\"#4dbeee\",\"port\":1,\"sid\":[\"\"],\"signalID\":32339,\"signalName\":\"Mux2\"},\"type\":\"RecordBlkView.Signal\",\"uuid\":\"\"},{\"content\":{\"blockPath\":[],\"channel\":[1],\"dimensions\":[6],\"domain\":\"\",\"lineColor\":\"#0072bd\",\"parentID\":32339,\"port\":1,\"sid\":[\"\"],\"signalID\":32340,\"signalName\":\"Mux2\"},\"t ...(+1236 chars)"  VisualizationBindings="{\"sparklinesplugin\":{\"info\":[{\"bindingParametersList\":[],\"subplotID\":1}]}}"
  Record7 : Record  FileSettingsInternal="{\"entries\":[{\"content\":{\"excelSettings\":{\"content\":{},\"type\":\"Streamout.ExcelSettings\"}},\"type\":\"Streamout.FileSettingStorage\",\"uuid\":\"\"}],\"packageUris\":[\"http:\\/\\/schema.mathworks.com\\/mf0\\/streamout_blocks\\/R2020a\"],\"version\":\"1.0\"}"  Layout=[1 1]  SignalsInternal="{\"entries\":[{\"content\":{\"signals\":[{\"content\":{\"blockPath\":[],\"dimensions\":[6,1],\"domain\":\"\",\"hasChildren\":true,\"lineColor\":\"#139fff\",\"port\":1,\"sid\":[\"\"],\"signalID\":32344,\"signalName\":\"Calculate Curve Errors:4\"},\"type\":\"RecordBlkView.Signal\",\"uuid\":\"\"},{\"content\":{\"blockPath\":[],\"channel\":[1,1],\"dimensions\":[6,1],\"domain\":\"\",\"lineColor\":\"#d95319\",\"parentID\":32344,\"port\":1,\"sid\":[\"\"],\"signalID\":323 ...(+1402 chars)"  VisualizationBindings="{\"sparklinesplugin\":{\"info\":[{\"bindingParametersList\":[],\"subplotID\":1}]}}"
  Record8 : Record  FileSettingsInternal="{\"entries\":[{\"content\":{\"excelSettings\":{\"content\":{},\"type\":\"Streamout.ExcelSettings\"}},\"type\":\"Streamout.FileSettingStorage\",\"uuid\":\"\"}],\"packageUris\":[\"http:\\/\\/schema.mathworks.com\\/mf0\\/streamout_blocks\\/R2020a\"],\"version\":\"1.0\"}"  Layout=[1 1]  SignalsInternal="{\"entries\":[{\"content\":{\"signals\":[{\"content\":{\"blockPath\":[],\"dimensions\":[6,1],\"domain\":\"\",\"hasChildren\":true,\"lineColor\":\"#b746ff\",\"port\":1,\"sid\":[\"\"],\"signalID\":32349,\"signalName\":\"Calculate Curve Errors:2\"},\"type\":\"RecordBlkView.Signal\",\"uuid\":\"\"},{\"content\":{\"blockPath\":[],\"channel\":[1,1],\"dimensions\":[6,1],\"domain\":\"\",\"lineColor\":\"#7e2f8e\",\"parentID\":32349,\"port\":1,\"sid\":[\"\"],\"signalID\":323 ...(+1402 chars)"  VisualizationBindings="{\"sparklinesplugin\":{\"info\":[{\"bindingParametersList\":[],\"subplotID\":1}]}}"
  S Block : Subsystem
  World Frame Control Force : Sum  Inputs=|++--
  Xd : Subsystem
  Control : Outport
  Curve E : Outport  Port=2
  wires:
  Reset Curve/1 -> S Block/8(Reset Curve)
  Eta 0-Order/1 -> S Block/4(Eta 0-Order)
  Eta 1-Order/1 -> S Block/5(Eta 1-Order)
  Body Velocities/1 -> Demux1/1, Fm/2(currentBodyrameVelocities)
  Calculate Curve Errors/2(EdotError) -> Record8/1, Edot/2(CurveErrorDot), S Block/2(curveErrorDot)
  mass/1 -> Xd/2(mass)
  Motion Curve Coefficents/1 -> Calculate Curve Errors/1(motionCurveCoefficents)
  currentPositionWorldFrame/1 -> Calculate World 2 Body Rotm/1(currentWorldFramePosition), Calculate Curve Errors/2(currentPositionWorldFrame)
  curveTime/1 -> Calculate Curve Errors/5(curveTime), S Block/3(curveTime)
  Xd/1(Motion Planner Control Force World Frame) -> World Frame Control Force/2, Record/1
  Calculate Curve Errors/1(EError) -> Curve E/1, S Block/1(curveError), Record4/1
  S Block/1("Sliding Mode Correction ") -> World Frame Control Force/3, Record1/1
  lamda/1 -> Edot/3(lamda), S Block/6(lamda)
  Rotational Inertias/1 -> Xd/3(Rotational Inertias)
  Calculate World 2 Body Rotm/1(world2Body) -> Body 2 World Rotm/1, Body2World/1, Edot/1(World2Body Rotm), S Block/7(World2Body Rotm), Xd/1(World2BodyRotm), Fm/1(world2BodyRotm)
  Edot/1(Curve Vel Correction) -> World Frame Control Force/4, Record2/1
  World Frame Control Force/1 -> Record5/1, Demux/1
  Demux/1 -> Mux/1
  Demux/2 -> Mux/2
  Demux/3 -> Mux/3
  Demux/6 -> Mux1/3
  Demux/5 -> Mux1/2
  Demux/4 -> Mux1/1
  Mux/1 -> Linear World To Body/2
  Mux1/1 -> Angular World To Body/2
  Linear World To Body/1 -> Mux2/1
  Angular World To Body/1 -> Mux2/2
  Mux2/1 -> Record6/1, Control/1
  Body2World/1 -> Angular World To Body/1, Linear World To Body/1
  Function Power/1 -> Calculate Curve Errors/7(functionPower)
  FunctionCount/1 -> Calculate Curve Errors/6(functionCount)
  tEst/1 -> Calculate Curve Errors/8(tEst)
  dragCoefficents/1 -> Fm/3(dragCoefficents)
  Body 2 World Rotm/1 -> Angular Velocities 2 Body Frame/1, Linear Velocities 2 Body Frame/1
  Linear Velocities 2 Body Frame/1 -> Mux3/1
  Angular Velocities 2 Body Frame/1 -> Mux3/2
  Mux3/1 -> Calculate Curve Errors/3(currentVelocityWorldFrame)
  Mux4/1 -> Linear Velocities 2 Body Frame/2
  Demux1/2 -> Mux4/2
  Demux1/1 -> Mux4/1
  Demux1/3 -> Mux4/3
  Demux1/5 -> Mux5/2
  Demux1/4 -> Mux5/1
  Demux1/6 -> Mux5/3
  Mux5/1 -> Angular Velocities 2 Body Frame/2
  setPoint/1 -> Calculate Curve Errors/4(setPoint)
  Fm/1(World Frame Drag Force) -> Record3/1, World Frame Control Force/1
  Calculate Curve Errors/3(EDoubleDot) -> Xd/4(Expected Accelerations)
  Calculate Curve Errors/4(curvePos) -> Record7/1

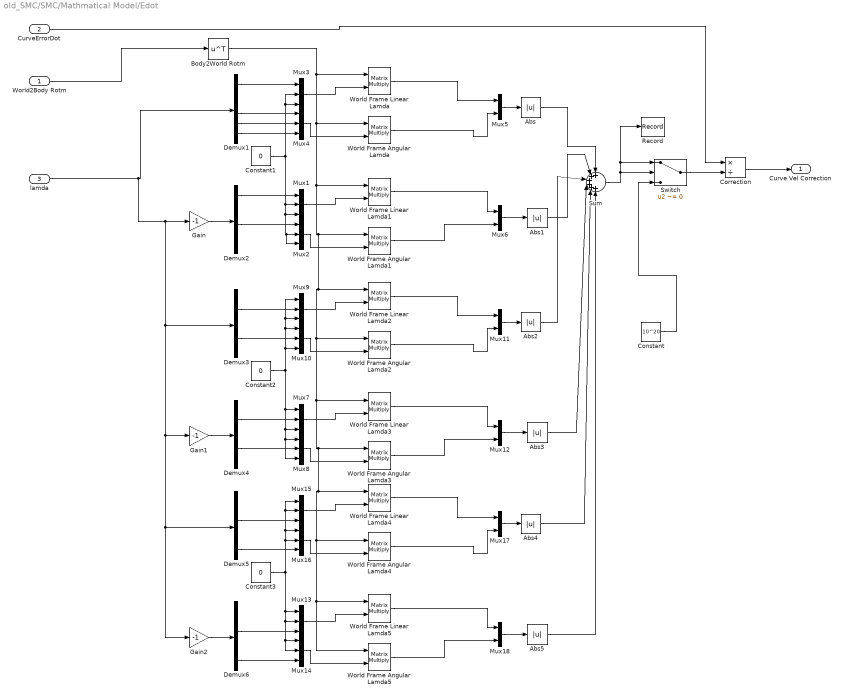
== system old_SMC/SMC/Mathmatical Model/Edot ==
  World2Body Rotm : Inport
  CurveErrorDot : Inport  Port=2
  lamda : Inport  Port=3
  Abs{,1..5} (6 alike) : Abs  SaturateOnIntegerOverflow=off
  Body2World Rotm : Math  Operator=transpose
  Constant : Constant  Value=10^20
  Constant1 : Constant  Value=0
  Constant2 : Constant  Value=0
  Constant3 : Constant  Value=0
  Correction : Product  Inputs=*/
  Demux{1..6} (6 alike) : Demux  Outputs=6
  Gain : Gain  Gain=-1
  Gain1 : Gain  Gain=-1
  Gain2 : Gain  Gain=-1
  Mux{1..4,7..10,13..16} (12 alike) : Mux  Inputs=3
  Mux{5..6,11..12,17..18} (6 alike) : Mux  Inputs=2
  Record : Record  FileSettingsInternal="{\"entries\":[{\"content\":{\"excelSettings\":{\"content\":{},\"type\":\"Streamout.ExcelSettings\"}},\"type\":\"Streamout.FileSettingStorage\",\"uuid\":\"\"}],\"packageUris\":[\"http:\\/\\/schema.mathworks.com\\/mf0\\/streamout_blocks\\/R2020a\"],\"version\":\"1.0\"}"  Layout=[1 1]  SignalsInternal="{\"entries\":[{\"content\":{\"signals\":[{\"content\":{\"blockPath\":[],\"dimensions\":[6],\"domain\":\"\",\"hasChildren\":true,\"lineColor\":\"#ff13a6\",\"port\":1,\"sid\":[\"\"],\"signalID\":32354,\"signalName\":\"Sum\"},\"type\":\"RecordBlkView.Signal\",\"uuid\":\"\"},{\"content\":{\"blockPath\":[],\"channel\":[1],\"dimensions\":[6],\"domain\":\"\",\"lineColor\":\"#4dbeee\",\"parentID\":32354,\"plots\":[1],\"port\":1,\"sid\":[\"\"],\"signalID\":32355,\"signalName\" ...(+1253 chars)"  VisualizationBindings="{\"sparklinesplugin\":{\"info\":[{\"bindingParametersList\":[],\"subplotID\":1}]}}"
  Sum : Sum  Inputs=++++++
  Switch : Switch  Criteria=u2 ~= 0  SaturateOnIntegerOverflow=off  InputSameDT=off
  World Frame Angular Lamda{,1..5} (6 alike) : Product  Multiplication=Matrix(*)
  World Frame Linear Lamda{,1..5} (6 alike) : Product  Multiplication=Matrix(*)
  Curve Vel Correction : Outport
  wires:
  Mux3/1 -> World Frame Linear Lamda/2
  CurveErrorDot/1 -> Correction/1
  World2Body Rotm/1 -> Body2World Rotm/1
  Mux4/1 -> World Frame Angular Lamda/2
  Demux1/4 -> Mux4/1
  Correction/1 -> Curve Vel Correction/1
  Demux1/1 -> Mux3/1
  Switch/1 -> Correction/2
  Constant/1 -> Switch/3
  Mux6/1 -> Abs1/1
  Sum/1 -> Record/1, Switch/1, Switch/2
  Mux5/1 -> Abs/1
  World Frame Linear Lamda/1 -> Mux5/1
  World Frame Angular Lamda/1 -> Mux5/2
  Demux2/1 -> Mux1/1
  Mux2/1 -> World Frame Angular Lamda1/2
  Mux1/1 -> World Frame Linear Lamda1/2
  World Frame Angular Lamda1/1 -> Mux6/2
  World Frame Linear Lamda1/1 -> Mux6/1
  Demux2/4 -> Mux2/1
  Demux1/5 -> Mux4/2
  Demux1/6 -> Mux4/3
  Gain/1 -> Demux2/1
  Constant1/1 -> Mux3/3, Mux3/2, Mux2/3, Mux2/2, Mux1/3, Mux1/2
  Abs/1 -> Sum/1
  Abs1/1 -> Sum/2
  Mux10/1 -> World Frame Angular Lamda2/2
  Mux8/1 -> World Frame Angular Lamda3/2
  World Frame Angular Lamda2/1 -> Mux11/2
  World Frame Angular Lamda3/1 -> Mux12/2
  Mux11/1 -> Abs2/1
  Constant2/1 -> Mux10/3, Mux10/1, Mux9/1, Mux9/3, Mux7/1, Mux8/3, Mux8/1, Mux7/3
  World Frame Linear Lamda3/1 -> Mux12/1
  Mux7/1 -> World Frame Linear Lamda3/2
  Demux4/5 -> Mux8/2
  Demux3/5 -> Mux10/2
  World Frame Linear Lamda2/1 -> Mux11/1
  Mux12/1 -> Abs3/1
  Mux9/1 -> World Frame Linear Lamda2/2
  Gain1/1 -> Demux4/1
  Mux16/1 -> World Frame Angular Lamda4/2
  Mux14/1 -> World Frame Angular Lamda5/2
  World Frame Angular Lamda4/1 -> Mux17/2
  lamda/1 -> Gain2/1, Demux5/1, Gain1/1, Demux3/1, Gain/1, Demux1/1
  World Frame Angular Lamda5/1 -> Mux18/2
  Mux17/1 -> Abs4/1
  Demux5/6 -> Mux16/3
  World Frame Linear Lamda5/1 -> Mux18/1
  Mux13/1 -> World Frame Linear Lamda5/2
  Body2World Rotm/1 -> World Frame Angular Lamda5/1, World Frame Linear Lamda5/1, World Frame Angular Lamda4/1, World Frame Linear Lamda4/1, World Frame Angular Lamda3/1, World Frame Linear Lamda3/1, World Frame Angular Lamda2/1, World Frame Linear Lamda2/1, World Frame Angular Lamda1/1, World Frame Linear Lamda1/1, World Frame Angular Lamda/1, World Frame Linear Lamda/1
  Demux6/6 -> Mux14/3
  World Frame Linear Lamda4/1 -> Mux17/1
  Mux18/1 -> Abs5/1
  Mux15/1 -> World Frame Linear Lamda4/2
  Gain2/1 -> Demux6/1
  Abs2/1 -> Sum/3
  Abs3/1 -> Sum/4
  Abs4/1 -> Sum/5
  Abs5/1 -> Sum/6
  Demux3/2 -> Mux9/2
  Demux4/2 -> Mux7/2
  Demux5/3 -> Mux15/3
  Demux6/3 -> Mux13/3
  Constant3/1 -> Mux16/2, Mux16/1, Mux15/1, Mux15/2, Mux13/1, Mux14/2, Mux14/1, Mux13/2

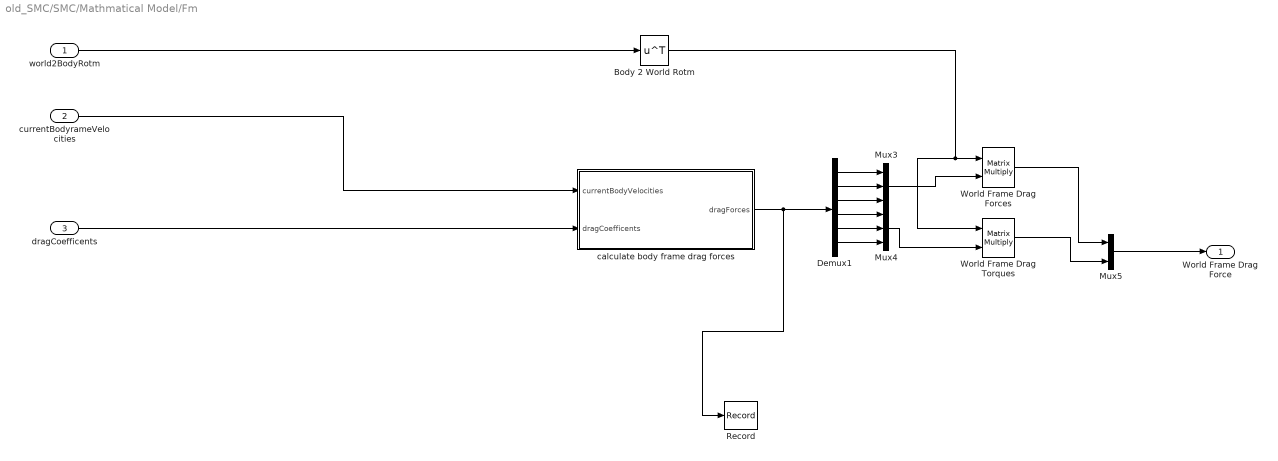
== system old_SMC/SMC/Mathmatical Model/Fm ==
  world2BodyRotm : Inport
  currentBodyrameVelocities : Inport  Port=2
  dragCoefficents : Inport  Port=3
  Body 2 World Rotm : Math  Operator=transpose
  Demux1 : Demux  Outputs=6
  Mux3 : Mux  Inputs=3
  Mux4 : Mux  Inputs=3
  Mux5 : Mux  Inputs=2
  Record : Record  FileSettingsInternal="{\"entries\":[{\"content\":{\"excelSettings\":{\"content\":{},\"type\":\"Streamout.ExcelSettings\"}},\"type\":\"Streamout.FileSettingStorage\",\"uuid\":\"\"}],\"packageUris\":[\"http:\\/\\/schema.mathworks.com\\/mf0\\/streamout_blocks\\/R2020a\"],\"version\":\"1.0\"}"  SignalsInternal="{\"entries\":[{\"content\":{\"signals\":[{\"content\":{\"blockPath\":[],\"dimensions\":[6,1],\"domain\":\"\",\"hasChildren\":true,\"lineColor\":\"#22b573\",\"port\":1,\"sid\":[\"\"],\"signalID\":32359,\"signalName\":\"calculate body frame drag forces\"},\"type\":\"RecordBlkView.Signal\",\"uuid\":\"\"},{\"content\":{\"blockPath\":[],\"channel\":[1,1],\"dimensions\":[6,1],\"domain\":\"\",\"lineColor\":\"#ff13a6\",\"parentID\":32359,\"plots\":[1],\"port\":1,\"sid\" ...(+1494 chars)"  VisualizationBindings="{\"sparklinesplugin\":{\"info\":[{\"bindingParametersList\":[],\"subplotID\":1}]}}"
  World Frame Drag Forces : Product  Multiplication=Matrix(*)
  World Frame Drag Torques : Product  Multiplication=Matrix(*)
  calculate body frame drag forces : MATLAB Function  TreatAsAtomicUnit=on
  World Frame Drag Force : Outport
  wires:
  World Frame Drag Forces/1 -> Mux5/1
  Demux1/4 -> Mux4/1
  Demux1/1 -> Mux3/1
  Mux3/1 -> World Frame Drag Forces/2
  Demux1/3 -> Mux3/3
  Demux1/6 -> Mux4/3
  Mux5/1 -> World Frame Drag Force/1
  Demux1/2 -> Mux3/2
  World Frame Drag Torques/1 -> Mux5/2
  currentBodyrameVelocities/1 -> calculate body frame drag forces/1(currentBodyVelocities)
  dragCoefficents/1 -> calculate body frame drag forces/2(dragCoefficents)
  Demux1/5 -> Mux4/2
  world2BodyRotm/1 -> Body 2 World Rotm/1
  Mux4/1 -> World Frame Drag Torques/2
  Body 2 World Rotm/1 -> World Frame Drag Torques/1, World Frame Drag Forces/1
  calculate body frame drag forces/1(dragForces) -> Record/1, Demux1/1

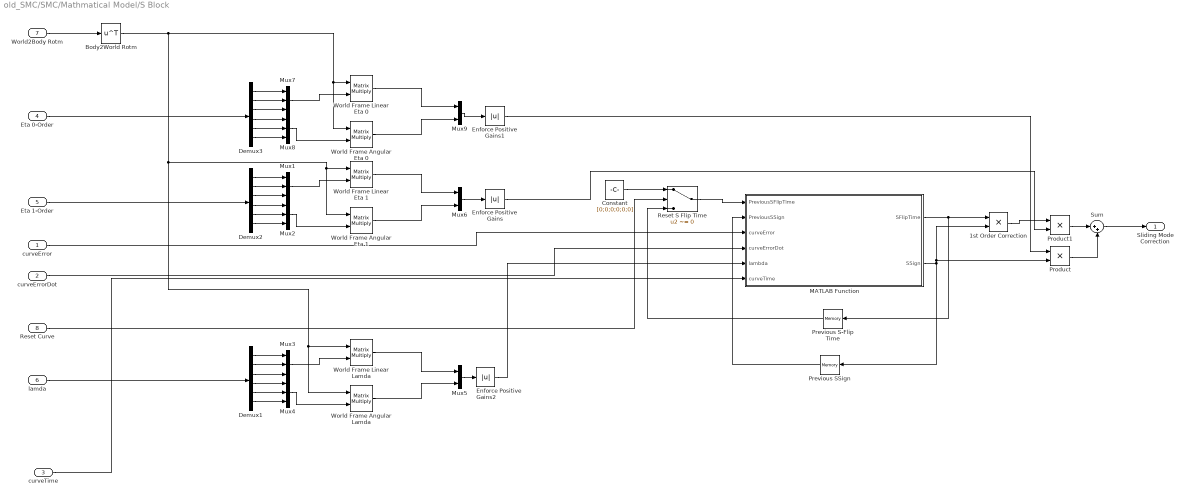
== system old_SMC/SMC/Mathmatical Model/S Block ==
  curveError : Inport
  curveErrorDot : Inport  Port=2
  curveTime : Inport  Port=3
  Eta 0-Order : Inport  Port=4
  Eta 1-Order : Inport  Port=5
  lamda : Inport  Port=6
  World2Body Rotm : Inport  Port=7
  Reset Curve : Inport  Port=8
  1st Order Correction : Product
  Body2World Rotm : Math  Operator=transpose
  Constant : Constant  Value=[0;0;0;0;0;0]
  Demux1 : Demux  Outputs=6
  Demux2 : Demux  Outputs=6
  Demux3 : Demux  Outputs=6
  Enforce Positive Gains : Abs  SaturateOnIntegerOverflow=off
  Enforce Positive Gains1 : Abs  SaturateOnIntegerOverflow=off
  Enforce Positive Gains2 : Abs  SaturateOnIntegerOverflow=off
  MATLAB Function : MATLAB Function  TreatAsAtomicUnit=on
  Mux{1..4,7..8} (6 alike) : Mux  Inputs=3
  Mux5 : Mux  Inputs=2
  Mux6 : Mux  Inputs=2
  Mux9 : Mux  Inputs=2
  Previous S-Flip Time : Memory  InitialCondition=[0;0;0;0;0;0]  InheritSampleTime=on
  Previous SSign : Memory  InitialCondition=[1;1;1;1;1;1]  InheritSampleTime=on
  Product : Product
  Product1 : Product
  Reset S Flip Time : Switch  Criteria=u2 ~= 0  SaturateOnIntegerOverflow=off  InputSameDT=off
  Sum : Sum  Inputs=|++
  World Frame Angular Eta 0 : Product  Multiplication=Matrix(*)
  World Frame Angular Eta 1 : Product  Multiplication=Matrix(*)
  World Frame Angular Lamda : Product  Multiplication=Matrix(*)
  World Frame Linear Eta 0 : Product  Multiplication=Matrix(*)
  World Frame Linear Eta 1 : Product  Multiplication=Matrix(*)
  World Frame Linear Lamda : Product  Multiplication=Matrix(*)
  "Sliding Mode Correction " : Outport
  wires:
  Previous SSign/1 -> MATLAB Function/2(PreviousSSign)
  Mux5/1 -> Enforce Positive Gains2/1
  MATLAB Function/2(SSign) -> 1st Order Correction/2, Product/2, Previous SSign/1
  curveTime/1 -> MATLAB Function/6(curveTime)
  MATLAB Function/1(SFlipTime) -> 1st Order Correction/1, Previous S-Flip Time/1
  curveErrorDot/1 -> MATLAB Function/4(curveErrorDot)
  curveError/1 -> MATLAB Function/3(curveError)
  Product/1 -> Sum/2
  Product1/1 -> Sum/1
  1st Order Correction/1 -> Product1/1
  Sum/1 -> "Sliding Mode Correction "/1
  Demux1/1 -> Mux3/1
  Demux1/2 -> Mux3/2
  lamda/1 -> Demux1/1
  Demux1/5 -> Mux4/2
  Demux1/3 -> Mux3/3
  Demux1/6 -> Mux4/3
  Mux3/1 -> World Frame Linear Lamda/2
  World Frame Linear Lamda/1 -> Mux5/1
  World Frame Angular Lamda/1 -> Mux5/2
  Demux1/4 -> Mux4/1
  Mux4/1 -> World Frame Angular Lamda/2
  Demux2/1 -> Mux1/1
  Demux2/4 -> Mux2/1
  Demux2/5 -> Mux2/2
  Demux2/2 -> Mux1/2
  Demux2/6 -> Mux2/3
  Demux2/3 -> Mux1/3
  World Frame Linear Eta 1/1 -> Mux6/1
  Mux1/1 -> World Frame Linear Eta 1/2
  Mux2/1 -> World Frame Angular Eta 1/2
  World Frame Angular Eta 1/1 -> Mux6/2
  Body2World Rotm/1 -> World Frame Linear Eta 1/1, World Frame Angular Eta 1/1, World Frame Linear Lamda/1, World Frame Angular Lamda/1, World Frame Angular Eta 0/1, World Frame Linear Eta 0/1
  Eta 1-Order/1 -> Demux2/1
  Mux6/1 -> Enforce Positive Gains/1
  Mux8/1 -> World Frame Angular Eta 0/2
  Demux3/2 -> Mux7/2
  Demux3/3 -> Mux7/3
  Eta 0-Order/1 -> Demux3/1
  Demux3/6 -> Mux8/3
  Demux3/1 -> Mux7/1
  Demux3/4 -> Mux8/1
  World Frame Linear Eta 0/1 -> Mux9/1
  Demux3/5 -> Mux8/2
  Mux9/1 -> Enforce Positive Gains1/1
  World Frame Angular Eta 0/1 -> Mux9/2
  Mux7/1 -> World Frame Linear Eta 0/2
  World2Body Rotm/1 -> Body2World Rotm/1
  Reset S Flip Time/1 -> MATLAB Function/1(PreviousSFlipTime)
  Previous S-Flip Time/1 -> Reset S Flip Time/3
  Constant/1 -> Reset S Flip Time/1
  Reset Curve/1 -> Reset S Flip Time/2
  Enforce Positive Gains/1 -> Product1/2
  Enforce Positive Gains1/1 -> Product/1
  Enforce Positive Gains2/1 -> MATLAB Function/5(lambda)

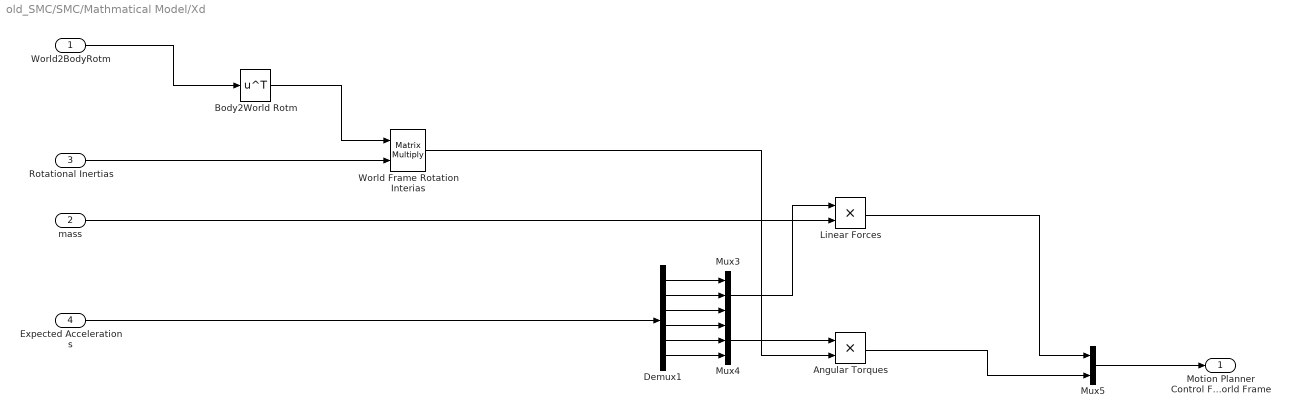
== system old_SMC/SMC/Mathmatical Model/Xd ==
  World2BodyRotm : Inport
  mass : Inport  Port=2
  Rotational Inertias : Inport  Port=3
  Expected Accelerations : Inport  Port=4
  Angular Torques : Product  Inputs=**
  Body2World Rotm : Math  Operator=transpose
  Demux1 : Demux  Outputs=6
  Linear Forces : Product  Inputs=**
  Mux3 : Mux  Inputs=3
  Mux4 : Mux  Inputs=3
  Mux5 : Mux  Inputs=2
  World Frame Rotation Interias : Product  Multiplication=Matrix(*)
  Motion Planner Control Force World Frame : Outport
  wires:
  Demux1/4 -> Mux4/1
  World2BodyRotm/1 -> Body2World Rotm/1
  Demux1/6 -> Mux4/3
  Demux1/5 -> Mux4/2
  Demux1/3 -> Mux3/3
  Demux1/2 -> Mux3/2
  Mux5/1 -> Motion Planner Control Force World Frame/1
  Demux1/1 -> Mux3/1
  Mux3/1 -> Linear Forces/1
  mass/1 -> Linear Forces/2
  Body2World Rotm/1 -> World Frame Rotation Interias/1
  Rotational Inertias/1 -> World Frame Rotation Interias/2
  Mux4/1 -> Angular Torques/1
  World Frame Rotation Interias/1 -> Angular Torques/2
  Angular Torques/1 -> Mux5/2
  Linear Forces/1 -> Mux5/1
  Expected Accelerations/1 -> Demux1/1

== matlab function old_SMC/SMC/Manage Curve Time ==
function curveTimeOffset = manageCurveTime(previousCurveTimeOffset, absoluteTime, resetCurveTime)

%reset one loop after curves are generated to avoid delay with curve
%generation
if(resetCurveTime)
    curveTimeOffset = absoluteTime;

    return
end

%keep previous if not reset
curveTimeOffset = previousCurveTimeOffset;

== matlab function old_SMC/SMC/Mathmatical Model/Calculate World 2 Body Rotm ==
function world2Body = fcn(currentWorldFramePosition)

%convert ros2 quat to matlab quat - quat is last 
quat = [currentWorldFramePosition(7), currentWorldFramePosition(4), currentWorldFramePosition(5), currentWorldFramePosition(6)];

%calculate the rotation matrix representing the current orientation
world2Body = quat2rotm(quat);

%matlab issue
world2Body = transpose(world2Body);

== matlab function old_SMC/SMC/Mathmatical Model/Fm/calculate body frame drag forces ==
function dragForces = fcn(currentBodyVelocities, dragCoefficents)

dragForces = zeros(6,1);

expectedDragCoefficentLength = 24;
if(expectedDragCoefficentLength ~= length(dragCoefficents))
    %drag coefficents are not the expected length
    return 
end

%reshape drag coefficents array into a more sensible form
dc = reshape(dragCoefficents, [expectedDragCoefficentLength / 6, 6]);

for i=1:6
    %calculate the forces created by drag
    dragForces(i) = dc(1, i) + abs(currentBodyVelocities(i)) * dc(2, i) + exp(abs(currentBodyVelocities(i)) / dc(4, i))* dc(3, i);

    %take into account sign
    sign = 0;
    if(currentBodyVelocities(i) ~= 0)
        sign = currentBodyVelocities(i) / abs(currentBodyVelocities(i));
    end

    dragForces(i) = sign * dragForces(i);
end

== matlab function old_SMC/SMC/Mathmatical Model/S Block/MATLAB Function ==
function [SFlipTime, SSign] = fcn(PreviousSFlipTime, PreviousSSign, curveError, curveErrorDot, lambda, curveTime)

%FlipTime, SSign and Previous are 6 by arrays - 1 per dof

SFlipTime = PreviousSFlipTime;
SSign = zeros(6,1);

%calculate S
S = curveError - lambda .* curveErrorDot;

%just so nothing explodes - ill be impressed if this happens
for i=1:6
    %ensure no S equals zero
    if(S(i) == 0)
        SSign(i) = 0;
    else
        SSign(i) = S(i) / abs(S(i));
    end
end

%see if S has flipped
for i=1:6
    if(SSign(i) * PreviousSSign(i) < 0)
        %S has flipped in dof i
        SFlipTime(i) = curveTime;
    end
end

== matlab function old_SMC/SMC/Mathmatical Model/Calculate Curve Errors ==
function [EError, EdotError, EDoubleDot, curvePos] = fcn(motionCurveCoefficents, currentPositionWorldFrame, currentVelocityWorldFrame, setPoint, curveTime, functionCount, functionPower, tEst)

%current position world frame and current velocity world frame are six * 1
%vectors

%default values
EError = zeros(6,1);
EdotError = zeros(6,1);
EDoubleDot = zeros(6,1);
curvePos = zeros(6,1);


if(tEst < 0)
    %there is no curve yet
    return
end

co = motionCurveCoefficents;
curveTimeNormalized = curveTime / tEst;

offsets = linspace(-pi(), pi() * (1 - 2 / functionCount), functionCount);

eulerOrientation = quat2eul([currentPositionWorldFrame(7),currentPositionWorldFrame(4),currentPositionWorldFrame(5),currentPositionWorldFrame(6)]);
eulerSetPoint = quat2eul([setPoint(7),setPoint(4),setPoint(5),setPoint(6)]);

currentPositionWorldFrameEuler = [currentPositionWorldFrame(1), currentPositionWorldFrame(2), currentPositionWorldFrame(3), eulerOrientation(1), eulerOrientation(2), eulerOrientation(3)];
setPointEuler = [setPoint(1), setPoint(2), setPoint(3), eulerSetPoint(1), eulerSetPoint(2), eulerSetPoint(3)];

%if in station keeping, calculate errors differently
if(curveTimeNormalized >= 1)
    for i= 1:6
        %each dof
    
        %calculate position error
        if(i <= 3)
            EError(i) = currentPositionWorldFrameEuler(i) - setPointEuler(i);
        else
            %for angular error - need to compensate for loop around
            EError(i) = currentPositionWorldFrameEuler(i) - setPointEuler(i);
    
            %normalize Error to 0 to 2pi
            EError(i) = mod(EError(i), 2 * pi());
    
            %if error greater than pi - smaller error in negative direction
            if(EError(i) > pi())
                EError(i) = EError(i) - 2 * pi();
            end
        end
    
        EdotError(i) = currentVelocityWorldFrame(i);
    end

    return
end

curvePos = zeros(6,1);
curveVel = zeros(6,1);

%evaulate each dof seperately
for i=1:6
    %calculate motion curve expected position
    curvePos(i) = 0;
    for j = 1:functionCount
        curvePos(i) = curvePos(i) + co(i, j) * sin(pi() / 2 * curveTimeNormalized + offsets(j)) ^ functionPower;
    end

    %calculate motion curve expected velocity
    curveVel(i) = 0;
    for j = 1:functionCount
        curveVel(i) = curveVel(i) + functionPower * co(i, j) / tEst * (pi() / 2 * sin(pi() / 2 * curveTimeNormalized + offsets(j)) ^ (functionPower - 1)) * cos(pi/2*curveTimeNormalized + offsets(j)); 
    end

    disp(currentPositionWorldFrameEuler(4))

    %calculate position error
    if(i <= 3)
        EError(i) = currentPositionWorldFrameEuler(i) - curvePos(i);
    else
        %for angular error - need to compensate for loop around
        EError(i) = currentPositionWorldFrameEuler(i) - curvePos(i);

        %normalize Error to 0 to 2pi
        EError(i) = mod(EError(i) + 2 * pi(), 2 * pi());

        %if error greater than pi - smaller error in negative direction
        if(EError(i) > pi())
            EError(i) = EError(i) - 2 * pi();
        end
    end

    %calculate velocity error
    EdotError(i) = currentVelocityWorldFrame(i) - curveVel(i);

    %calculate desired acceleration
    for j = 1:functionCount
        EDoubleDot(i) = EDoubleDot(i) + functionPower * co(i, j) / (tEst^2) * pi()^2 / 4 * (cos(pi()/2 * curveTimeNormalized + offsets(j))^2 *(functionPower - 1) * sin(pi()/2 * curveTimeNormalized + offsets(j))^(functionPower - 2) - sin(pi()/2* curveTimeNormalized + offsets(j))^functionPower); 
    end
end
